simulink model "sfun_03"  (R2018b)
settings: Solver=VariableStepAuto  StartTime=0.0  StopTime=10.0  RelTol=1e-3
settings Model: Creator=student  LastModifiedBy=student

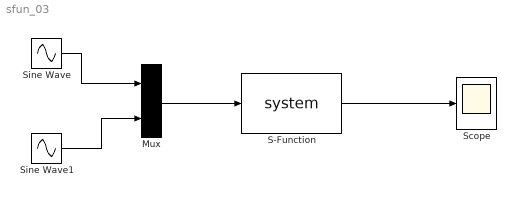
== system sfun_03 ==
  Mux : Mux  Inputs=2
  S-Function : S-Function  SFunctionDeploymentMode=off  EnableBusSupport=off
  Scope : Scope
  Sine Wave : Sin  SampleTime=0
  Sine Wave1 : Sin  SampleTime=0
  wires:
  Sine Wave1/1 -> Mux/2
  Sine Wave/1 -> Mux/1
  S-Function/1 -> Scope/1
  Mux/1 -> S-Function/1
